simulink model "two_phase_main_loop"  (R2025b)
settings: Solver=ode23t  StartTime=0.0  StopTime=CFG.t_stop  RelTol=1e-3
undefined symbols (not defined in the file): cfg, CFG, u_cmd
libraries: fl_lib x21, nesl_utility x20, SimscapeFluids_lib x6
(part 2 of 2)

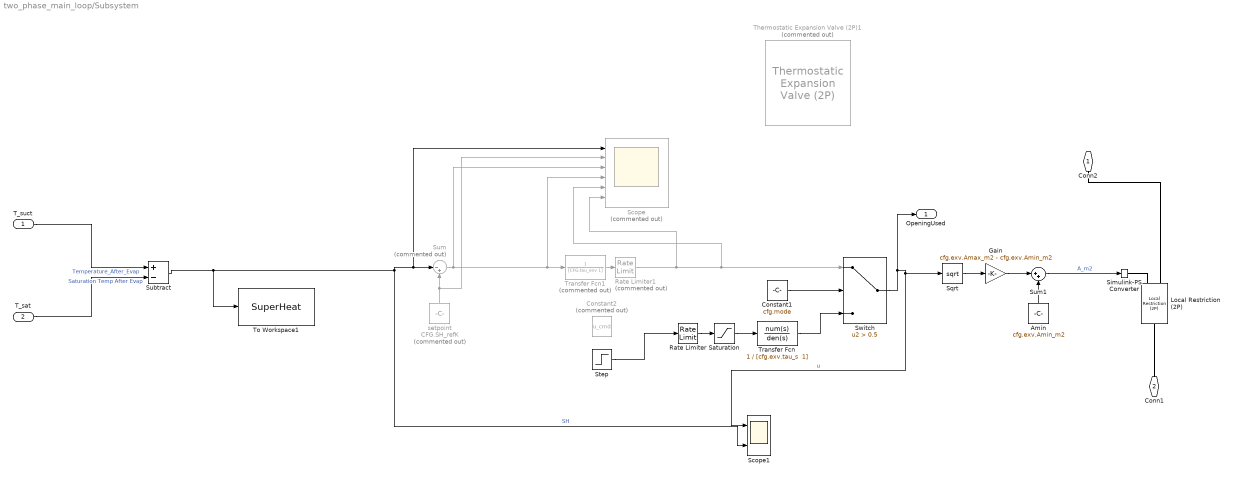
== system two_phase_main_loop/Subsystem ==
  T_suct : Inport
  T_sat : Inport  Port=2
  Amin : Constant  Value=cfg.exv.Amin_m2
  Constant1 : Constant  Value=cfg.mode
  Constant2 : Constant  Commented=on  Value=u_cmd
  Gain : Gain  Gain=cfg.exv.Amax_m2 - cfg.exv.Amin_m2
  Local Restriction (2P) : fl_lib/Two-Phase Fluid/Elements/Local Restriction (2P)  restriction_type=foundation.enum.restriction_type.variable  restriction_area=1e-3 m^2  min_area="cfg.exv.Amin_m2  m^2"  max_area="cfg.exv.Amax_m2  m^2"  pressure_loss_model=foundation.enum.RestrictionPressureLossModel.Bernoulli  area=pi*0.02^2/4 m^2  Cd=0.64  B_lam=0.999
      settings: InternalSimscapePortConfiguration="{\"Bottom\":[],\"Left\":[{\"id\":\"A\",\"label\":\"A\",\"type\":\"foundation.two_phase_fluid.two_phase_fluid\"},{\"id\":\"area_in\",\"label\":\"AR\",\"type\":\"input\"}],\"Right\":[{\"id\":\"B\",\"label\":\"B\",\"type\":\"foundation.two_phase_fluid.two_phase_fluid\"}],\"Top\":[]}"
  Rate Limiter : RateLimiter  RisingSlewLimit=cfg.exv.rate_lim_per_s  FallingSlewLimit=- cfg.exv.rate_lim_per_s  SampleTimeMode=inherited  LinearizeAsGain=off
  Rate Limiter1 : RateLimiter  Commented=on  RisingSlewLimit=CFG.rate_lim  FallingSlewLimit=-CFG.rate_lim  SampleTimeMode=inherited  InitialCondition=CFG.Opening_init
  Saturation : Saturate  UpperLimit=cfg.exv.u_max  LowerLimit=cfg.exv.u_min
  Scope : Scope  Commented=on  NumInputPorts=6
      settings: ActiveDisplayYMinimum=-103.41458668465931  ActiveDisplayYMaximum=76.487544358108849  DataLoggingVariableName=ScopeData2
  Scope1 : Scope  NumInputPorts=2
      settings: ActiveDisplayYMinimum=-0.54056692529291384  ActiveDisplayYMaximum=1.3123579665285228  DataLoggingVariableName=ScopeData3
  Simulink-PS Converter : nesl_utility/Simulink-PS Converter  PhysicalDomain=network_engine_domain  SubClassName=ps_input  LeftPortType=input  RightPortType=output  PseudoPeriodic=off  Frequencies=[]  NoiseDistribution=none  NoiseParameters=[]  Unit=m^2  AffineConversion=off  FilteringAndDerivatives=provide  SimscapeFilterOrder=1  InputFilterTimeConstant=0.001  UdotUserProvided=0
  Sqrt : Sqrt
  Step : Step  Time=cfg.exv.step_time_s  Before=cfg.exv.step_u1  After=cfg.exv.step_u2  SampleTime=0
  Subtract : Sum  Inputs=+-
  Sum : Sum  Commented=on  Inputs=|-+
  Sum1 : Sum  Inputs=|++
  Switch : Switch  Criteria=u2 > Threshold  Threshold=0.5  SaturateOnIntegerOverflow=off  InputSameDT=off
  Thermostatic Expansion Valve (2P)1 : SimscapeFluids_lib/Two-Phase Fluid/Valves & Orifices/Flow Control Valves/Thermostatic Expansion Valve (2P)  Commented=on  valve_parameterization=fluids.two_phase_fluid.valves_orifices.flow_control_valves.enum.ThermostaticExpansionValveParameterization.Nominal  capacity_spec=fluids.two_phase_fluid.valves_orifices.flow_control_valves.enum.ThermostaticExpansionValveCapacitySpec.HeatTransfer  Q_nominal=16 kW  Q_max=16 * 1.5 kW  mdot_nominal=0.005 kg/s  mdot_max=0.008 kg/s  pressure_spec=fluids.two_phase_fluid.valves_orifices.flow_control_valves.enum.ThermostaticExpansionValvePressureSpec.SaturationTemperature  p_cond_nominal=1.5 MPa  p_evap_nominal=0.5 MPa  T_cond_nominal=45 degC  T_evap_nominal=5 degC  delta_T_sub=5 deltaK  delta_T_nominal=5 deltaK  delta_T_static=2 deltaK  mop=fluids.two_phase_fluid.valves_orifices.flow_control_valves.enum.ThermostaticExpansionValveMOP.Off  p_mop=0.5 MPa  T_mop=288.15 K  T_evap_out_TLU1=0 : 10 : 40 degC  p_bulb_TLU1=0.3 : 0.1 : 0.7 MPa  lift_TLU2=0 : 0.15 : 0.6 mm  p_evap_TLU2=0.3 : -0.05 : 0.1 MPa  lift_TLU3=0 : 0.15 : 0.6 mm  mdot_TLU3=0 : 0.015 : 0.06 kg/s  p_cond_ref=2 MPa  p_evap_ref=0.2 MPa  T_evap_out_ref=0 degC  delta_T_sub_ref=5 deltaK  pressure_equalization=fluids.two_phase_fluid.valves_orifices.flow_control_valves.enum.ThermostaticExpansionValveEqualization.Internal  bulb_dynamics=simscape.enum.onoff.off  tau_bulb=20 s  leakage_fraction=1e-6  smoothing_factor=0.01  B_lam=0.999  tau_x=0.1 s  area=pi*0.02^2/4 m^2
      settings: InternalSimscapePortConfiguration="{\"Bottom\":[],\"Left\":[{\"id\":\"A\",\"label\":\"A\",\"type\":\"foundation.two_phase_fluid.two_phase_fluid\"}],\"Right\":[{\"id\":\"B\",\"label\":\"B\",\"type\":\"foundation.two_phase_fluid.two_phase_fluid\"}],\"Top\":[{\"id\":\"S\",\"label\":\"S\",\"type\":\"foundation.two_phase_fluid.two_phase_fluid\"}]}"
  To Workspace1 : ToWorkspace  VariableName=SuperHeat  SampleTime=-1
  Transfer Fcn : TransferFcn  Numerator=1  Denominator="[cfg.exv.tau_s  1]"
  Transfer Fcn1 : TransferFcn  Commented=on  Numerator=1  Denominator=[CFG.tau_exv 1]
  setpoint : Constant  Commented=on  Value=CFG.SH_refK
  Conn2 : PMIOPort  Side=Left
  Conn1 : PMIOPort  Port=2  Side=Right
  OpeningUsed : Outport
  wires:
  Transfer Fcn1/1 -> Rate Limiter1/1
  Switch/1 -> OpeningUsed/1, Sqrt/1, Scope1/1  "u"
  Rate Limiter1/1 -> Scope/5, Switch/1, Scope/6
  Constant1/1 -> Switch/2
  Sum/1 -> Transfer Fcn1/1, Scope/4, Scope/3
  Rate Limiter/1 -> Saturation/1
  Transfer Fcn/1 -> Switch/3
  Subtract/1 -> Scope1/2, Sum/1, Scope/1, To Workspace1/1  "SH"
  Saturation/1 -> Transfer Fcn/1
  setpoint/1 -> Sum/2, Scope/2
  Sum1/1 -> Simulink-PS Converter/1  "A_m2"
  T_suct/1 -> Subtract/1  "Temperature_After_Evap"
  T_sat/1 -> Subtract/2  "Saturation Temp After Evap"
  Sqrt/1 -> Gain/1
  Gain/1 -> Sum1/1
  Amin/1 -> Sum1/2
  Step/1 -> Rate Limiter/1
  connections:
  Local Restriction (2P)/LConn1 -- Conn2/RConn1
  Local Restriction (2P)/RConn1 -- Conn1/RConn1
  Simulink-PS Converter/RConn1 -- Local Restriction (2P)/LConn2

== matlab function two_phase_main_loop/Calculation: mdot˙(hout​−hin​)/MATLAB Function ==
  data: h_in_kJpkg input; ton output; h_out_kJpkg input; mdot_kgps input
function ton = calc_tonnage(h_in_kJpkg, h_out_kJpkg, mdot_kgps)
%   calc_tonnage  Computes system capacity in refrigeration tons.
%
%   ton = calc_tonnage(h_in_kJpkg, h_out_kJpkg, mdot_kgps, mode)
%
%   Inputs
%   -------
%   h_in_kJpkg   : inlet specific enthalpy  [kJ/kg]
%   h_out_kJpkg  : outlet specific enthalpy [kJ/kg]
%   mdot_kgps    : mass flow rate           [kg/s]
%
%   Output
%   -------
%   ton          : capacity in refrigeration tons [TR]
%
%   Notes
%   -----
%   • For evaporators (cooling): Q̇ = ṁ × (h_out − h_in)
%   • 1 ton refrigeration = 3.517 kW
%
%   Example
%   -------
%       ton_cool = calc_tonnage(250, 430, 0.05);
%


Qdot_kW = mdot_kgps .* (h_out_kJpkg - h_in_kJpkg); % kJ/kg × kg/s = kJ/s = kW


ton = Qdot_kW ./ 3.517; % Convert to refrigeration tons

end
